simulink model "swap_model"  (R2025b)
settings: Solver=FixedStepAuto  StartTime=0.0  StopTime=50  FixedStep=0.01  RelTol=1e-3
model workspace (MAT data in the model file):
  D_normal = 100
  D_spare = 100
  D_total = 200
  S = 16000000
  buf_per_blocked = 4
  epsilon = 0.05
  f = 100000
libraries: simulink x1
settings Model: Creator=aalpar  LastModifiedBy=aalpar

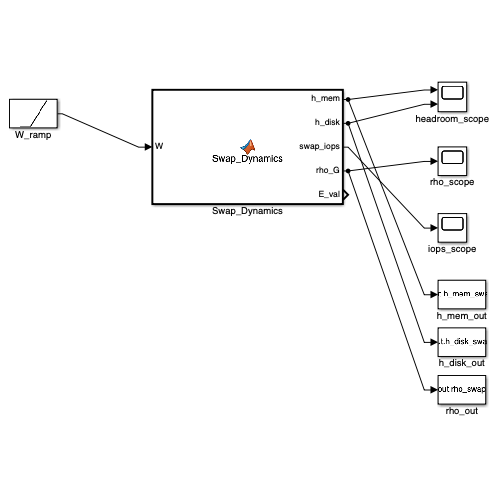
[thumbnail: Simulink's stored preview of the top-level diagram]
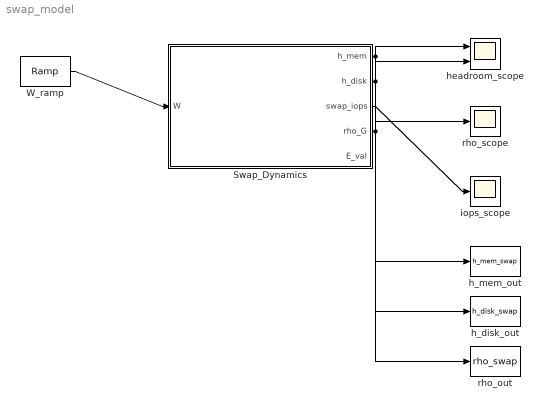
== system swap_model ==
  Swap_Dynamics : MATLAB Function  TreatAsAtomicUnit=on
  W_ramp : simulink/Sources/Ramp  slope=16000  start=0  InitialOutput=15984000
  h_disk_out : ToWorkspace  VariableName=h_disk_swap  SaveFormat=Timeseries  SampleTime=-1
  h_mem_out : ToWorkspace  VariableName=h_mem_swap  SaveFormat=Timeseries  SampleTime=-1
  headroom_scope : Scope  NumInputPorts=2
  iops_scope : Scope
  rho_out : ToWorkspace  VariableName=rho_swap  SaveFormat=Timeseries  SampleTime=-1
  rho_scope : Scope
  wires:
  W_ramp/1 -> Swap_Dynamics/1(W)
  Swap_Dynamics/1(h_mem) -> headroom_scope/1, h_mem_out/1
  Swap_Dynamics/2(h_disk) -> headroom_scope/2, h_disk_out/1
  Swap_Dynamics/4(rho_G) -> rho_scope/1, rho_out/1
  Swap_Dynamics/3(swap_iops) -> iops_scope/1

== matlab function swap_model/Swap_Dynamics ==
  data: W input; h_mem output; h_disk output; swap_iops output; rho_G output; E_val output
function [h_mem, h_disk, swap_iops, rho_G, E_val] = Swap_Dynamics(W)
% Cross-resource swap feedback dynamics.
S = 1.6e+07; f = 100000;
D_total = 200; D_normal = 100; D_spare = 100;
eps_ = 0.05; buf_per_blocked = 4;

% Excess working set
E_val = max(0, W - S);

% Page fault rate and swap IOPS
if W > 0
    fault_prob = E_val / W;
else
    fault_prob = 0;
end
swap_iops = 2 * f * fault_prob;  % 2 IOPS per fault (in + out)

% Headroom
h_mem = S - (W - E_val);  % pages of memory headroom (simplified)
h_disk = D_spare - swap_iops;

% Gain matrix
alpha = 2 * f / max(W, 1);       % d(swap_IOPS)/d(-h_mem)
beta = buf_per_blocked * 0.001;   % d(mem_demand)/d(-h_disk)
G = [eps_, beta; alpha, eps_];
rho_G = max(abs(eig(G)));
